simulink model "Simulation_sliding_mode_control_single_rank_inverted_pendulum"  (R2023a)
settings: Solver=VariableStepAuto  StartTime=0.0  StopTime=10.0  RelTol=1e-3
settings Model: Creator=ACCENT  LastModifiedBy=ACCENT

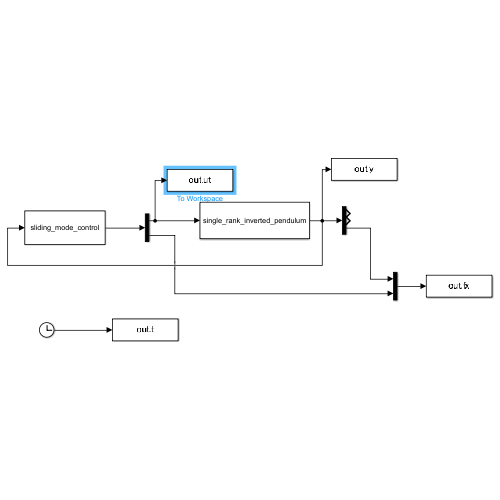
[thumbnail: Simulink's stored preview of the top-level diagram]
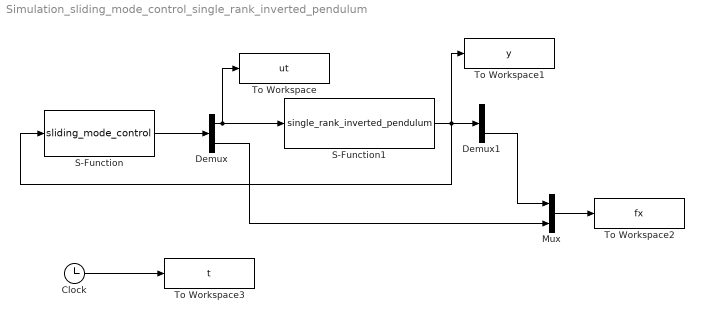
== system Simulation_sliding_mode_control_single_rank_inverted_pendulum ==
  Clock : Clock
      settings: Decimation=30
  Demux : Demux  Outputs=2
  Demux1 : Demux  Outputs=3
  Mux : Mux  Inputs=2
  S-Function : S-Function  FunctionName=sliding_mode_control  SFunctionDeploymentMode=off  EnableBusSupport=off
  S-Function1 : S-Function  FunctionName=single_rank_inverted_pendulum  SFunctionDeploymentMode=off  EnableBusSupport=off
  To Workspace : ToWorkspace  VariableName=ut  SampleTime=-1
  To Workspace1 : ToWorkspace  VariableName=y  SampleTime=-1
  To Workspace2 : ToWorkspace  VariableName=fx  SampleTime=-1
  To Workspace3 : ToWorkspace  VariableName=t  SampleTime=-1
  wires:
  S-Function/1 -> Demux/1
  Demux/1 -> S-Function1/1, To Workspace/1
  S-Function1/1 -> To Workspace1/1, S-Function/1, Demux1/1
  Demux1/3 -> Mux/1
  Demux/2 -> Mux/2
  Mux/1 -> To Workspace2/1
  Clock/1 -> To Workspace3/1
